simulink model "TJA_StateMachine"  (R2018b)
settings: Solver=VariableStepAuto  StartTime=0.0  StopTime=10.0  RelTol=1e-3
libraries: simulink x2
settings Model: Creator=石丽  LastModifiedBy=石丽

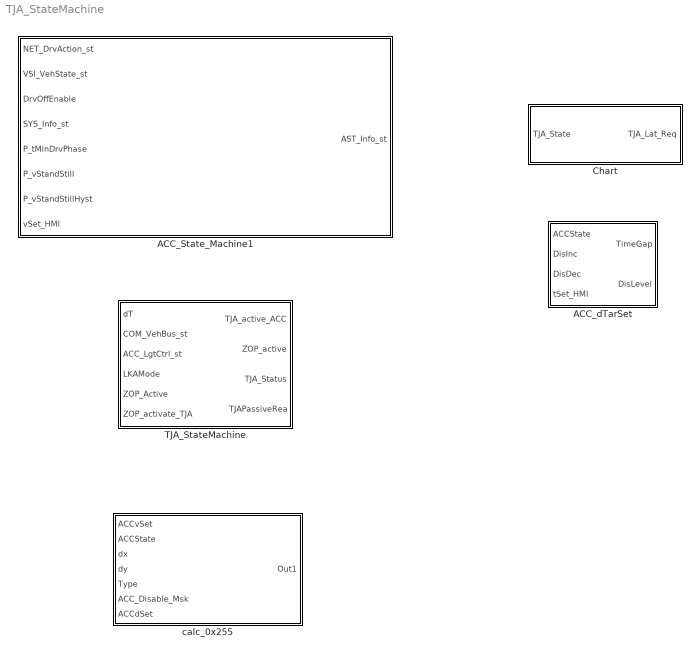
== system TJA_StateMachine ==
  ACC_State_Machine1 : Stateflow chart  TreatAsAtomicUnit=on
  ACC_dTarSet : Subsystem
  Chart : Stateflow chart  TreatAsAtomicUnit=on
  TJA_StateMachine : Subsystem
  calc_0x255 : Subsystem

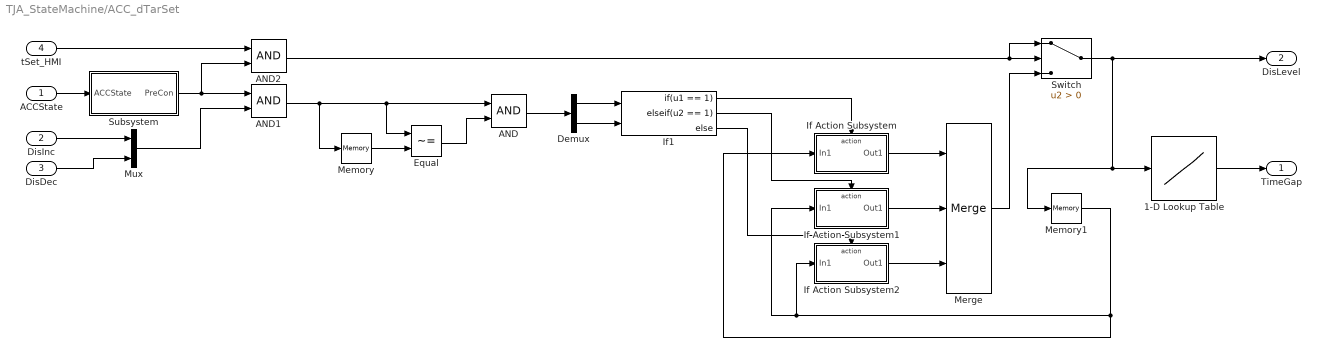
== system TJA_StateMachine/ACC_dTarSet ==
  ACCState : Inport
  DisInc : Inport  Port=2
  DisDec : Inport  Port=3
  tSet_HMI : Inport  Port=4
  1-D Lookup Table : Lookup_n-D  NumberOfTableDimensions=1  BreakpointsForDimension1=[1 2 3]  Table=[1.2 1.8 2.1]  InterpMethod=Flat  InternalRulePriority=Speed  RndMeth=Simplest  InputSameDT=on
  AND : Logic  AllPortsSameDT=off  OutDataTypeStr=boolean
  AND1 : Logic  AllPortsSameDT=off  OutDataTypeStr=boolean
  AND2 : Logic  AllPortsSameDT=off  OutDataTypeStr=boolean
  Demux : Demux  Outputs=2
  Equal : RelationalOperator  Operator=~=  OutDataTypeStr=boolean  RndMeth=Simplest
  If Action Subsystem : Subsystem  TreatAsAtomicUnit=on
  If Action Subsystem1 : Subsystem  TreatAsAtomicUnit=on
  If Action Subsystem2 : Subsystem  TreatAsAtomicUnit=on
  If1 : If  NumInputs=2  IfExpression=u1 == 1  ElseIfExpressions=u2 == 1
  Memory : Memory
  Memory1 : Memory  InitialCondition=3
  Merge : Merge  Inputs=3  InitialOutput=0
  Mux : Mux  Inputs=2
  Subsystem : Subsystem
  Switch : Switch  Criteria=u2 > Threshold
  TimeGap : Outport
  DisLevel : Outport  Port=2
  wires:
  If1/1 -> If Action Subsystem/Action
  If Action Subsystem/1(Out1) -> Merge/1
  Memory1/1 -> If Action Subsystem/1(In1), If Action Subsystem1/1(In1), If Action Subsystem2/1(In1)
  If Action Subsystem1/1(Out1) -> Merge/2
  If1/2 -> If Action Subsystem1/Action
  If Action Subsystem2/1(Out1) -> Merge/3
  If1/3 -> If Action Subsystem2/Action
  Subsystem/1(PreCon) -> AND2/2, AND1/1
  AND1/1 -> Memory/1, Equal/1, AND/1
  Memory/1 -> Equal/2
  Equal/1 -> AND/2
  AND/1 -> Demux/1
  Demux/1 -> If1/1
  Demux/2 -> If1/2
  Mux/1 -> AND1/2
  ACCState/1 -> Subsystem/1(ACCState)
  DisInc/1 -> Mux/1
  DisDec/1 -> Mux/2
  1-D Lookup Table/1 -> TimeGap/1
  Switch/1 -> DisLevel/1, Memory1/1, 1-D Lookup Table/1
  Merge/1 -> Switch/3
  tSet_HMI/1 -> AND2/1
  AND2/1 -> Switch/1, Switch/2

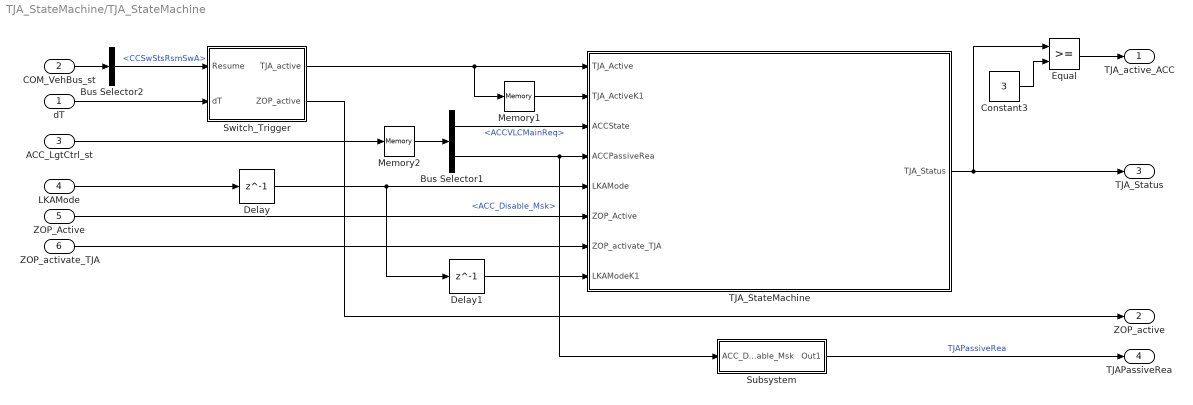
== system TJA_StateMachine/TJA_StateMachine ==
  dT : Inport
  COM_VehBus_st : Inport  Port=2
  ACC_LgtCtrl_st : Inport  Port=3
  LKAMode : Inport  Port=4
  ZOP_Active : Inport  Port=5
  ZOP_activate_TJA : Inport  Port=6
  Bus Selector1 : BusSelector  OutputSignals=ACCVLCMainReq,ACC_Disable_Msk
  Bus Selector2 : BusSelector  OutputSignals=x1E1.CCSwStsRsmSwA
  Constant3 : Constant  Value=3  OutDataTypeStr=single
  Delay : Delay  DelayLength=1
  Delay1 : Delay  DelayLength=1
  Equal : RelationalOperator  OutDataTypeStr=boolean  RndMeth=Simplest
  Memory1 : Memory
  Memory2 : Memory
  Subsystem : Subsystem
  Switch_Trigger : Subsystem
  TJA_StateMachine : Stateflow chart  TreatAsAtomicUnit=on
  TJA_active_ACC : Outport
  ZOP_active : Outport  Port=2
  TJA_Status : Outport  Port=3
  TJAPassiveRea : Outport  Port=4
  wires:
  Switch_Trigger/1(TJA_active) -> Memory1/1, TJA_StateMachine/1(TJA_Active)
  Bus Selector1/1 -> TJA_StateMachine/3(ACCState)  "<ACCVLCMainReq>"
  Switch_Trigger/2(ZOP_active) -> ZOP_active/1
  Memory2/1 -> Bus Selector1/1
  COM_VehBus_st/1 -> Bus Selector2/1
  Bus Selector1/2 -> Subsystem/1(ACC_Disable_Msk), TJA_StateMachine/4(ACCPassiveRea)  "<ACC_Disable_Msk>"
  dT/1 -> Switch_Trigger/2(dT)
  Bus Selector2/1 -> Switch_Trigger/1(Resume)  "<CCSwStsRsmSwA>"
  Memory1/1 -> TJA_StateMachine/2(TJA_ActiveK1)
  ACC_LgtCtrl_st/1 -> Memory2/1
  TJA_StateMachine/1(TJA_Status) -> Equal/1, TJA_Status/1
  Constant3/1 -> Equal/2
  Equal/1 -> TJA_active_ACC/1
  LKAMode/1 -> Delay/1
  ZOP_Active/1 -> TJA_StateMachine/6(ZOP_Active)
  ZOP_activate_TJA/1 -> TJA_StateMachine/7(ZOP_activate_TJA)
  Subsystem/1(Out1) -> TJAPassiveRea/1  "TJAPassiveRea"
  Delay/1 -> Delay1/1, TJA_StateMachine/5(LKAMode)
  Delay1/1 -> TJA_StateMachine/8(LKAModeK1)

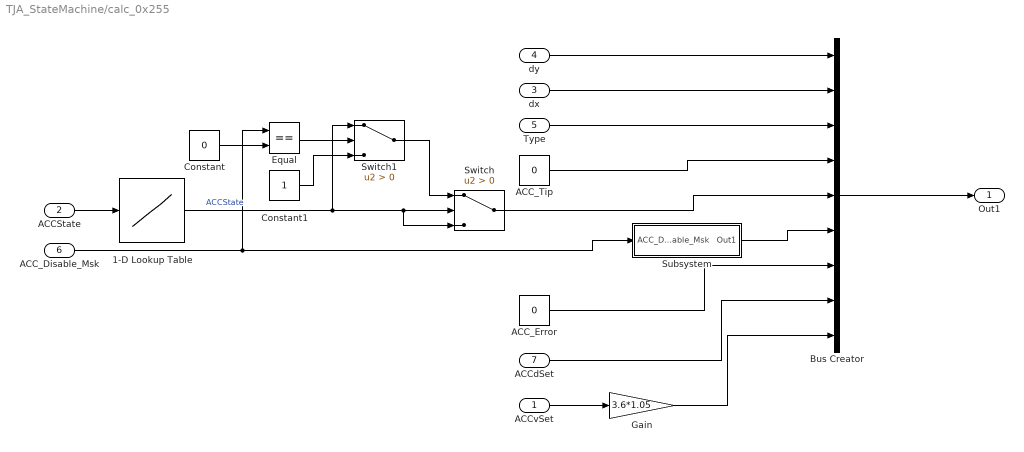
== system TJA_StateMachine/calc_0x255 ==
  ACCvSet : Inport
  ACCState : Inport  Port=2
  dx : Inport  Port=3
  dy : Inport  Port=4
  Type : Inport  Port=5
  ACC_Disable_Msk : Inport  Port=6
  ACCdSet : Inport  Port=7
  1-D Lookup Table : Lookup_n-D  NumberOfTableDimensions=1  BreakpointsForDimension1=[0,1,2,3,4]  Table=[0,2,3,3,4]  InterpMethod=Flat  InternalRulePriority=Speed  RndMeth=Simplest  InputSameDT=on
  ACC_Error : Constant  Value=0  OutDataTypeStr=single
  ACC_Tip : Constant  Value=0  OutDataTypeStr=single
  Bus Creator : BusCreator  Inputs=9  OutDataTypeStr=Bus: x255  NonVirtualBus=on
      settings: InheritFromInputs=off
  Constant : Constant  Value=0
  Constant1 : Constant
  Equal : RelationalOperator  Operator===  OutDataTypeStr=boolean  RndMeth=Simplest
  Gain : Gain  Gain=3.6*1.05
  Subsystem : Subsystem
  Switch : Switch  Criteria=u2 > Threshold  OutDataTypeStr=single
  Switch1 : Switch  Criteria=u2 > Threshold
  Out1 : Outport
  wires:
  dy/1 -> Bus Creator/1
  dx/1 -> Bus Creator/2
  Type/1 -> Bus Creator/3
  ACC_Tip/1 -> Bus Creator/4
  ACCState/1 -> 1-D Lookup Table/1
  ACC_Error/1 -> Bus Creator/7
  ACCdSet/1 -> Bus Creator/8
  ACCvSet/1 -> Gain/1
  Bus Creator/1 -> Out1/1
  Subsystem/1(Out1) -> Bus Creator/6
  ACC_Disable_Msk/1 -> Subsystem/1(ACC_Disable_Msk), Equal/1
  Gain/1 -> Bus Creator/9
  1-D Lookup Table/1 -> Switch1/1, Switch/2, Switch/3  "ACCState"
  Switch/1 -> Bus Creator/5
  Constant/1 -> Equal/2
  Equal/1 -> Switch1/2
  Switch1/1 -> Switch/1
  Constant1/1 -> Switch1/3

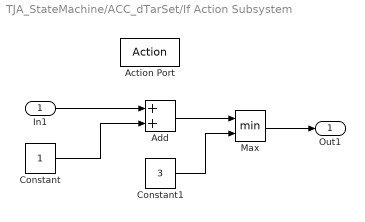
== system TJA_StateMachine/ACC_dTarSet/If Action Subsystem ==
  In1 : Inport
  Action Port : ActionPort
  Add : Sum
  Constant : Constant  OutDataTypeStr=single
  Constant1 : Constant  Value=3  OutDataTypeStr=single
  Max : MinMax  Inputs=2
  Out1 : Outport
  wires:
  In1/1 -> Add/1
  Constant/1 -> Add/2
  Max/1 -> Out1/1
  Add/1 -> Max/1
  Constant1/1 -> Max/2

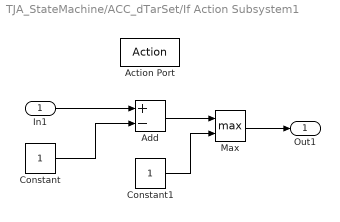
== system TJA_StateMachine/ACC_dTarSet/If Action Subsystem1 ==
  In1 : Inport
  Action Port : ActionPort
  Add : Sum  Inputs=+-
  Constant : Constant  OutDataTypeStr=single
  Constant1 : Constant  OutDataTypeStr=single
  Max : MinMax  Function=max  Inputs=2
  Out1 : Outport
  wires:
  In1/1 -> Add/1
  Constant/1 -> Add/2
  Add/1 -> Max/1
  Max/1 -> Out1/1
  Constant1/1 -> Max/2

== system TJA_StateMachine/ACC_dTarSet/If Action Subsystem2 ==
  In1 : Inport
  Action Port : ActionPort
  Out1 : Outport
  wires:
  In1/1 -> Out1/1

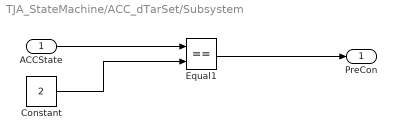
== system TJA_StateMachine/ACC_dTarSet/Subsystem ==
  ACCState : Inport
  Constant : Constant  Value=2  OutDataTypeStr=single
  Equal1 : RelationalOperator  Operator===  OutDataTypeStr=boolean  RndMeth=Simplest
  PreCon : Outport
  wires:
  Constant/1 -> Equal1/2
  ACCState/1 -> Equal1/1
  Equal1/1 -> PreCon/1

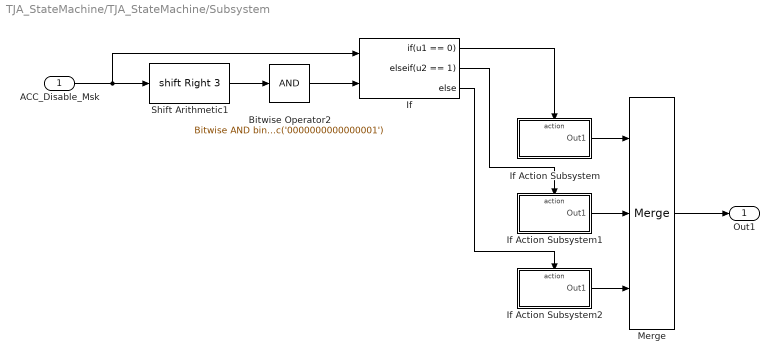
== system TJA_StateMachine/TJA_StateMachine/Subsystem ==
  ACC_Disable_Msk : Inport
  Bitwise Operator2 : simulink/Logic and Bit Operations/Bitwise Operator  logicop=AND  UseBitMask=on  BitMask=bin2dec('0000000000000001')  BitMaskRealWorld=Stored Integer
  If : If  NumInputs=2  IfExpression=u1 == 0  ElseIfExpressions=u2 == 1
  If Action Subsystem : Subsystem  TreatAsAtomicUnit=on
  If Action Subsystem1 : Subsystem  TreatAsAtomicUnit=on
  If Action Subsystem2 : Subsystem  TreatAsAtomicUnit=on
  Merge : Merge  Inputs=3
  Shift Arithmetic1 : ArithShift  BitShiftNumber=3  BitShiftDirection=Right
  Out1 : Outport
  wires:
  If Action Subsystem/1(Out1) -> Merge/1
  If/3 -> If Action Subsystem2/Action
  Bitwise Operator2/1 -> If/2
  Shift Arithmetic1/1 -> Bitwise Operator2/1
  If/1 -> If Action Subsystem/Action
  If Action Subsystem2/1(Out1) -> Merge/3
  If/2 -> If Action Subsystem1/Action
  Merge/1 -> Out1/1
  If Action Subsystem1/1(Out1) -> Merge/2
  ACC_Disable_Msk/1 -> If/1, Shift Arithmetic1/1

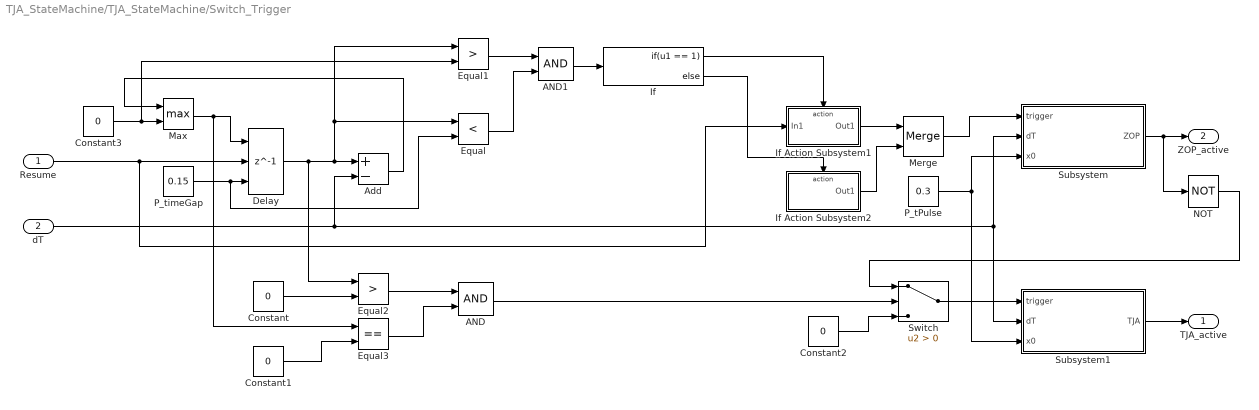
== system TJA_StateMachine/TJA_StateMachine/Switch_Trigger ==
  Resume : Inport
  dT : Inport  Port=2
  AND : Logic  AllPortsSameDT=off  OutDataTypeStr=boolean
  AND1 : Logic  AllPortsSameDT=off  OutDataTypeStr=boolean
  Add : Sum  Inputs=+-
  Constant : Constant  Value=0
  Constant1 : Constant  Value=0
  Constant2 : Constant  Value=0
  Constant3 : Constant  Value=0  OutDataTypeStr=single
  Delay : Delay  DelayLength=1  InitialConditionSource=Input port  ExternalReset=Falling
      settings: InputPortMap=u0,r5,p4
  Equal : RelationalOperator  Operator=<  OutDataTypeStr=boolean  RndMeth=Simplest
  Equal1 : RelationalOperator  Operator=>  OutDataTypeStr=boolean  RndMeth=Simplest
  Equal2 : RelationalOperator  Operator=>  OutDataTypeStr=boolean  RndMeth=Simplest
  Equal3 : RelationalOperator  Operator===  OutDataTypeStr=boolean  RndMeth=Simplest
  If : If  IfExpression=u1 == 1
  If Action Subsystem1 : Subsystem  TreatAsAtomicUnit=on
  If Action Subsystem2 : Subsystem  TreatAsAtomicUnit=on
  Max : MinMax  Function=max  Inputs=2
  Merge : Merge
  NOT : Logic  Operator=NOT  AllPortsSameDT=off  OutDataTypeStr=boolean
  P_tPulse : Constant  Value=0.3
  P_timeGap : Constant  Value=0.15
  Subsystem : Subsystem
  Subsystem1 : Subsystem
  Switch : Switch  Criteria=u2 > Threshold
  TJA_active : Outport
  ZOP_active : Outport  Port=2
  wires:
  Delay/1 -> Equal2/1, Equal1/1, Equal/1, Add/1
  Max/1 -> Equal3/1, Delay/1
  Constant3/1 -> Equal1/2, Max/2
  Add/1 -> Max/1
  Resume/1 -> If Action Subsystem1/1(In1), Delay/2
  P_timeGap/1 -> Equal/2, Delay/3
  Equal1/1 -> AND1/1
  AND1/1 -> If/1
  If/1 -> If Action Subsystem1/Action
  dT/1 -> Subsystem1/2(dT), Subsystem/2(dT), Add/2
  If Action Subsystem2/1(Out1) -> Merge/2
  If Action Subsystem1/1(Out1) -> Merge/1
  If/2 -> If Action Subsystem2/Action
  Subsystem/1(ZOP) -> NOT/1, ZOP_active/1
  Subsystem1/1(TJA) -> TJA_active/1
  Merge/1 -> Subsystem/1(trigger)
  P_tPulse/1 -> Subsystem1/3(x0), Subsystem/3(x0)
  Equal/1 -> AND1/2
  Constant/1 -> Equal2/2
  Constant1/1 -> Equal3/2
  Equal2/1 -> AND/1
  Equal3/1 -> AND/2
  AND/1 -> Switch/2
  Switch/1 -> Subsystem1/1(trigger)
  Constant2/1 -> Switch/3
  NOT/1 -> Switch/1

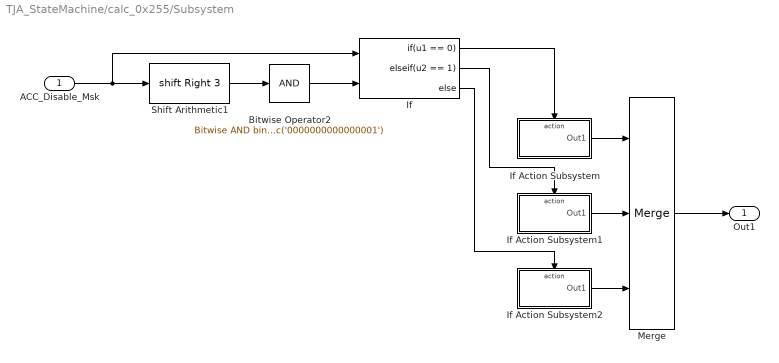
== system TJA_StateMachine/calc_0x255/Subsystem ==
  ACC_Disable_Msk : Inport
  Bitwise Operator2 : simulink/Logic and Bit Operations/Bitwise Operator  logicop=AND  UseBitMask=on  BitMask=bin2dec('0000000000000001')  BitMaskRealWorld=Stored Integer
  If : If  NumInputs=2  IfExpression=u1 == 0  ElseIfExpressions=u2 == 1
  If Action Subsystem : Subsystem  TreatAsAtomicUnit=on
  If Action Subsystem1 : Subsystem  TreatAsAtomicUnit=on
  If Action Subsystem2 : Subsystem  TreatAsAtomicUnit=on
  Merge : Merge  Inputs=3
  Shift Arithmetic1 : ArithShift  BitShiftNumber=3  BitShiftDirection=Right
  Out1 : Outport
  wires:
  If Action Subsystem/1(Out1) -> Merge/1
  If/3 -> If Action Subsystem2/Action
  Bitwise Operator2/1 -> If/2
  Shift Arithmetic1/1 -> Bitwise Operator2/1
  If/1 -> If Action Subsystem/Action
  If Action Subsystem2/1(Out1) -> Merge/3
  If/2 -> If Action Subsystem1/Action
  Merge/1 -> Out1/1
  If Action Subsystem1/1(Out1) -> Merge/2
  ACC_Disable_Msk/1 -> If/1, Shift Arithmetic1/1

== system TJA_StateMachine/TJA_StateMachine/Subsystem/If Action Subsystem ==
  Action Port : ActionPort
  Constant : Constant  Value=0  OutDataTypeStr=single
  Out1 : Outport
  wires:
  Constant/1 -> Out1/1

== system TJA_StateMachine/TJA_StateMachine/Subsystem/If Action Subsystem1 ==
  Action Port : ActionPort
  Constant : Constant  Value=4  OutDataTypeStr=single
  Out1 : Outport
  wires:
  Constant/1 -> Out1/1

== system TJA_StateMachine/TJA_StateMachine/Subsystem/If Action Subsystem2 ==
  Action Port : ActionPort
  Constant : Constant  Value=5  OutDataTypeStr=single
  Out1 : Outport
  wires:
  Constant/1 -> Out1/1

== system TJA_StateMachine/TJA_StateMachine/Switch_Trigger/If Action Subsystem1 ==
  In1 : Inport
  Action Port : ActionPort
  Out1 : Outport
  wires:
  In1/1 -> Out1/1

== system TJA_StateMachine/TJA_StateMachine/Switch_Trigger/If Action Subsystem2 ==
  Action Port : ActionPort
  Constant : Constant  Value=0  OutDataTypeStr=boolean
  Out1 : Outport
  wires:
  Constant/1 -> Out1/1

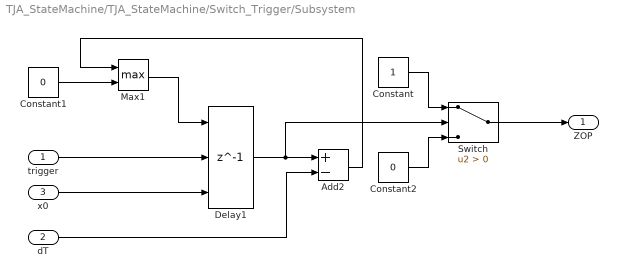
== system TJA_StateMachine/TJA_StateMachine/Switch_Trigger/Subsystem ==
  trigger : Inport
  dT : Inport  Port=2
  x0 : Inport  Port=3
  Add2 : Sum  Inputs=+-
  Constant : Constant
  Constant1 : Constant  Value=0
  Constant2 : Constant  Value=0
  Delay1 : Delay  DelayLength=1  InitialConditionSource=Input port  ExternalReset=Rising
      settings: InputPortMap=u0,r5,p4
  Max1 : MinMax  Function=max  Inputs=2
  Switch : Switch  Criteria=u2 > Threshold
  ZOP : Outport
  wires:
  Max1/1 -> Delay1/1
  Delay1/1 -> Switch/2, Add2/1
  x0/1 -> Delay1/3
  Constant/1 -> Switch/1
  trigger/1 -> Delay1/2
  Constant1/1 -> Max1/2
  Constant2/1 -> Switch/3
  dT/1 -> Add2/2
  Add2/1 -> Max1/1
  Switch/1 -> ZOP/1

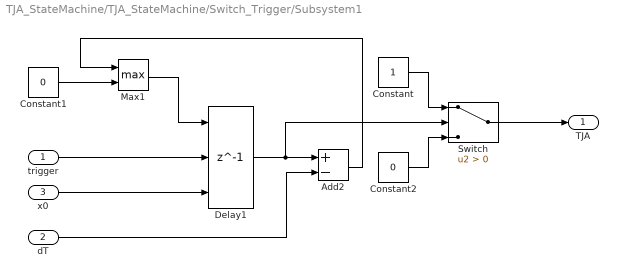
== system TJA_StateMachine/TJA_StateMachine/Switch_Trigger/Subsystem1 ==
  trigger : Inport
  dT : Inport  Port=2
  x0 : Inport  Port=3
  Add2 : Sum  Inputs=+-
  Constant : Constant
  Constant1 : Constant  Value=0
  Constant2 : Constant  Value=0
  Delay1 : Delay  DelayLength=1  InitialConditionSource=Input port  ExternalReset=Rising
      settings: InputPortMap=u0,r5,p4
  Max1 : MinMax  Function=max  Inputs=2
  Switch : Switch  Criteria=u2 > Threshold
  TJA : Outport
  wires:
  Max1/1 -> Delay1/1
  Delay1/1 -> Switch/2, Add2/1
  x0/1 -> Delay1/3
  Constant/1 -> Switch/1
  trigger/1 -> Delay1/2
  Constant1/1 -> Max1/2
  Constant2/1 -> Switch/3
  dT/1 -> Add2/2
  Add2/1 -> Max1/1
  Switch/1 -> TJA/1

== system TJA_StateMachine/calc_0x255/Subsystem/If Action Subsystem ==
  Action Port : ActionPort
  Constant : Constant  Value=0  OutDataTypeStr=single
  Out1 : Outport
  wires:
  Constant/1 -> Out1/1

== system TJA_StateMachine/calc_0x255/Subsystem/If Action Subsystem1 ==
  Action Port : ActionPort
  Constant : Constant  Value=4  OutDataTypeStr=single
  Out1 : Outport
  wires:
  Constant/1 -> Out1/1

== system TJA_StateMachine/calc_0x255/Subsystem/If Action Subsystem2 ==
  Action Port : ActionPort
  Constant : Constant  Value=5  OutDataTypeStr=single
  Out1 : Outport
  wires:
  Constant/1 -> Out1/1

== stateflow chart TJA_StateMachine/ACC_State_Machine1 ==
  note: MainState
      | 0	OFF
      | 1	PASSIVE
      | 2	ACTIVE_Drive
      | 3	ACTIVE_Standstill
      | 4	OVERRIDE
  state OFF
    en:
    AST_Info_st.MainState = 0;
    AST_Info_st.tMinInDrv = 0;
    AST_Info_st.vSet = 0;
  state OVERRIDE
    en:
    AST_Info_st.MainState = 4;
    AST_Info_st.tMinInDrv = 0;
  state PASSIVE
    en:
    AST_Info_st.MainState = 1;
    AST_Info_st.tMinInDrv = 0;
  state ACTIVE
    en:
    if ((NET_DrvAction_st.ACC_SetSw == 1)&&(NET_DrvAction_st.ACC_SetSwK1 == 0))
    AST_Info_st.vSet = round(VSI_VehState_st.vRef*1.05*3.6)/1.05/3.6;
    end
    AST_Info_st.vSet = min(AST_Info_st.vSet, (120/1.05)/3.6);
    AST_Info_st.vSet = max(AST_Info_st.vSet, (30/1.05)/3.6);
    du:
    if ((NET_DrvAction_st.ACC_SpdIncSw == 1)&&(NET_DrvAction_st.ACC_SpdIncSwK1 == 0))
    AST_Info_st.vSet = AST_Info_st.vSet + (5 - mod(round(AST_Info_st.vSet*1.05*3.6),5))/1.05/3.6;
    else if ((NET_DrvAction_st.ACC_SpdDecSw == 1)&&(NET_DrvAction_st.ACC_SpdDecSwK1 == 0))
    AST_Info_st.vSet = AST_Info_st.vSet + (mod(5 - mod(round(AST_Info_st.vSet*1.05*3.6),5),5))/1.05/3.6 - 5/1.05/3.6;
    end
    end
    if (vSet_HMI.vSetAccSpd ~= 0)
    AST_Info_st.vSet = vSet_HMI.vSetAccSpd/1.05/3.6;
    end
    AST_Info_st.vSet = min(AST_Info_st.vSet, (120/1.05)/3.6);
    AST_Info_st.vSet = max(AST_Info_st.vSet, (30/1.05)/3.6);
    state Drive
      en:
      AST_Info_st.MainState = 2;
      du:
      if(VSI_VehState_st.vRef > P_vStandStillHyst)
      if(AST_Info_st.tMinInDrv > SYS_Info_st.dT)
      AST_Info_st.tMinInDrv = AST_Info_st.tMinInDrv - SYS_Info_st.dT;
      else
      AST_Info_st.tMinInDrv = 0;
      end
      end
    state Standstill
      en:
      AST_Info_st.MainState = 3;
      AST_Info_st.tMinInDrv = P_tMinDrvPhase;
    (default) -> Drive
    Drive -> Standstill : [VSI_VehState_st.vRef < P_vStandStill...
        | &&AST_Info_st.tMinInDrv == 0]
    Standstill -> Drive : [DrvOffEnable == 1]
  (default) -> OFF
  OVERRIDE -> OFF [order 3] : [NET_DrvAction_st.ACC_MainSw == 0]
  ACTIVE -> OFF [order 3] : [NET_DrvAction_st.ACC_MainSw == 0]
  OVERRIDE -> PASSIVE [order 2] : [NET_DrvAction_st.ACC_CancelSw == 1||NET_DrvAction_st.BrakePedalApply == 1||NET_DrvAction_st.GearLever < 3]
  ACTIVE -> OVERRIDE [order 1] : [NET_DrvAction_st.DrvOverride == 1]
  OVERRIDE -> ACTIVE [order 1] : [NET_DrvAction_st.DrvOverride == 0]
  OFF -> PASSIVE : [NET_DrvAction_st.ACC_MainSw == 1]
  PASSIVE -> OFF [order 2] : [NET_DrvAction_st.ACC_MainSw == 0]
  PASSIVE -> ACTIVE [order 1] : [(NET_DrvAction_st.ACC_SetSw == 1||(NET_DrvAction_st.ACC_ResSw == 1&&AST_Info_st.vSet ~= 0))&&NET_DrvAction_st.BrakePedalApply == 0&&NET_DrvAction_st.GearLever >= 3]
  ACTIVE -> PASSIVE [order 2] : [NET_DrvAction_st.ACC_CancelSw == 1||NET_DrvAction_st.BrakePedalApply == 1||NET_DrvAction_st.GearLever < 3]
  data: NET_DrvAction_st input; AST_Info_st output Bus: AST_INFO_ST; VSI_VehState_st input; DrvOffEnable input; SYS_Info_st input; P_tMinDrvPhase input; P_vStandStill input; P_vStandStillHyst input; vSet_HMI input Bus: ACC_HMI_REQ

== stateflow chart TJA_StateMachine/TJA_StateMachine ==
  note: TJA_Status:
      | 0 Off
      | 1 Passive
      | 2 Standby
      | 3 Active
      | 4 Override
      | 5 Error
  note: ACCState:
      | 0 Off
      | 1 Passive
      | 2 Drive
      | 3 Standstill
      | 4 Override
  state Off
    en:
    TJA_Status = 0;
  state Passive
    en:
    TJA_Status = 1;
  state Standby
    en:
    TJA_Status = 2;
  note: LKAMode:
      | 0 Error
      | 1 Off
      | 2 Idle
      | 3 Ready
      | 4 Active
  state Error
    en:
    TJA_Status = 5;
  state Override
    en:
    TJA_Status = 4;
  state Active
    en:
    TJA_Status = 3;
  Off -> Standby [order 3] : [ACCState == 1 && ACCPassiveRea == 0 && LKAMode == 3]
  Standby -> Off [order 3] : [ACCState == 0 || LKAMode == 1]
  (default) -> Off
  Off -> Passive [order 1] : [ACCState == 1 && LKAMode ==2]
  Passive -> Standby [order 1] : [ACCPassiveRea == 0 && LKAMode == 3]
  Passive -> Off [order 2] : [ACCState == 0 || LKAMode == 1]
  Standby -> Passive [order 2] : [ACCPassiveRea ~= 0 || LKAMode == 2]
  Passive -> Error [order 3] : [LKAMode == 0]
  Active -> Passive [order 2] : [ACCPassiveRea ~= 0 || LKAMode == 2]
  Standby -> Error [order 4] : [LKAMode == 0]
  Error -> Off : [LKAMode == 1]
  Off -> Error [order 2] : [LKAMode == 0]
  Override -> Off [order 3] : [ACCState == 0 || LKAMode == 1]
  Active -> Off [order 3] : [ACCState == 0 || LKAMode == 1]
  Override -> Passive [order 2] : [ACCPassiveRea ~= 0 || LKAMode == 2]
  Override -> Standby [order 5] : [LKAModeK1 >= 4 && LKAMode == 3]
  Active -> Standby [order 5] : [ZOP_Active == 1 || (LKAModeK1 >= 4 && LKAMode == 3)]
  Standby -> Active [order 1] : [(TJA_Active == 1 && TJA_ActiveK1 == 0 && ZOP_Active == 0) || ZOP_activate_TJA == 1]
  Active -> Override [order 1] : [ACCState == 4]
  Override -> Error [order 4] : [LKAMode == 0]
  Override -> Active [order 1] : [ACCState == 3 || ACCState == 2]
  Active -> Error [order 4] : [LKAMode == 0]
  data: TJA_Status output; TJA_Active input; TJA_ActiveK1 input; ACCState input; ACCPassiveRea input; LKAMode input; ZOP_Active input; ZOP_activate_TJA input; LKAModeK1 input

== stateflow chart TJA_StateMachine/Chart ==
  state TJA_Lat_Req_Reset
    en:
    TJA_Lat_Req=0;
  state TJA_Lat_Req_Set
    en:
    TJA_Lat_Req=1;
  (default) -> TJA_Lat_Req_Reset
  TJA_Lat_Req_Reset -> TJA_Lat_Req_Set : [TJA_State == 3]
  TJA_Lat_Req_Set -> TJA_Lat_Req_Reset : [TJA_State < 3 || TJA_State == 5]
  data: TJA_State input; TJA_Lat_Req output double
